simulink model "pidsimu"  (Simulink 6.0)
settings: Solver=ode45  StartTime=0.0  StopTime=60  MaxStep=1  MinStep=0.001  RelTol=1e-2
settings Model: LastModifiedBy=hp  BufferReuse=off
settings SolverCC: InitialStep=0.01
settings DataIOCC: SignalLoggingName=sigsOut  Refine=3
settings OptimizationCC: InlineInvariantSignals=off  OptimizeBlockIOStorage=off  BufferReuse=off  EnforceIntegerDowncast=off  ExpressionFolding=off  FoldNonRolledExpr=off  LocalBlockOutputs=off
settings DebuggingCC: SolverPrmCheckMsg=none
settings HardwareCC: TargetUnknown=on

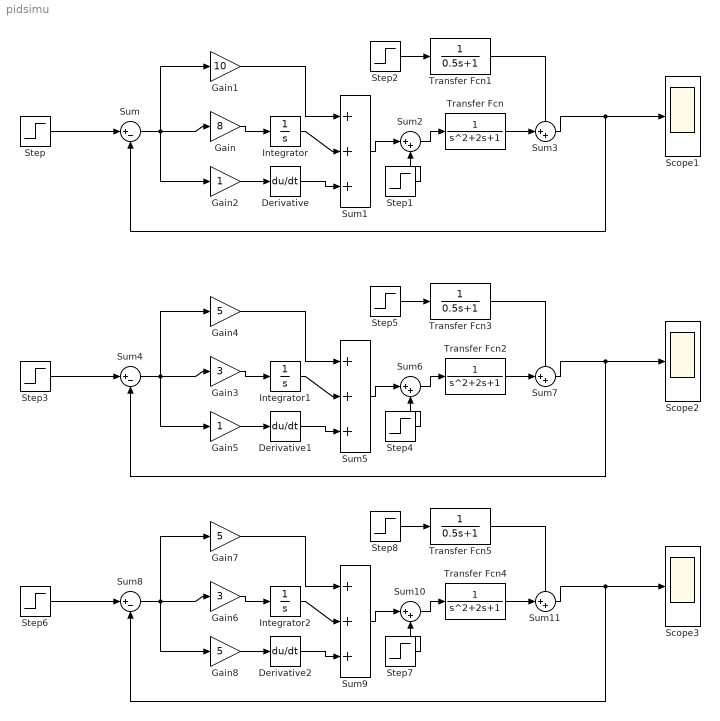
== system pidsimu ==
  Derivative : Derivative
  Derivative1 : Derivative
  Derivative2 : Derivative
  Gain : Gain  Gain=8  SaturateOnIntegerOverflow=on
  Gain1 : Gain  Gain=10  SaturateOnIntegerOverflow=on
  Gain2 : Gain  SaturateOnIntegerOverflow=on
  Gain3 : Gain  Gain=3  SaturateOnIntegerOverflow=on
  Gain4 : Gain  Gain=5  SaturateOnIntegerOverflow=on
  Gain5 : Gain  SaturateOnIntegerOverflow=on
  Gain6 : Gain  Gain=3  SaturateOnIntegerOverflow=on
  Gain7 : Gain  Gain=5  SaturateOnIntegerOverflow=on
  Gain8 : Gain  Gain=5  SaturateOnIntegerOverflow=on
  Integrator : Integrator
  Integrator1 : Integrator
  Integrator2 : Integrator
  Scope1 : Scope
      settings: TimeRange=60  YMin=0  YMax=1.5  SampleInput=on
  Scope2 : Scope
      settings: TimeRange=60  YMin=0  YMax=1.5  SampleInput=on
  Scope3 : Scope
      settings: TimeRange=60  YMin=0  YMax=1.5  SaveName=ScopeData2  SampleInput=on
  Step : Step  Time=0  SampleTime=0.1
  Step1 : Step  Time=20  SampleTime=0.1
  Step2 : Step  Time=40  SampleTime=0.1
  Step3 : Step  Time=0  SampleTime=0.1
  Step4 : Step  Time=20  SampleTime=0.1
  Step5 : Step  Time=40  SampleTime=0.1
  Step6 : Step  Time=0  SampleTime=0.1
  Step7 : Step  Time=20  SampleTime=0.1
  Step8 : Step  Time=40  SampleTime=0.1
  Sum : Sum  Inputs=|+-  SaturateOnIntegerOverflow=on
  Sum1 : Sum  Inputs=|+++  SaturateOnIntegerOverflow=on
  Sum{2..3,6..7,10..11} (6 alike) : Sum  Inputs=|++  SaturateOnIntegerOverflow=on
  Sum4 : Sum  Inputs=|+-  SaturateOnIntegerOverflow=on
  Sum5 : Sum  Inputs=|+++  SaturateOnIntegerOverflow=on
  Sum8 : Sum  Inputs=|+-  SaturateOnIntegerOverflow=on
  Sum9 : Sum  Inputs=|+++  SaturateOnIntegerOverflow=on
  Transfer Fcn : TransferFcn  Numerator=[1 ]
  Transfer Fcn1 : TransferFcn  Numerator=[1 ]  Denominator=[ 0.5 1]
  Transfer Fcn2 : TransferFcn  Numerator=[1 ]
  Transfer Fcn3 : TransferFcn  Numerator=[1 ]  Denominator=[ 0.5 1]
  Transfer Fcn4 : TransferFcn  Numerator=[1 ]
  Transfer Fcn5 : TransferFcn  Numerator=[1 ]  Denominator=[ 0.5 1]
  wires:
  Step/1 -> Sum/1
  Sum/1 -> Gain/1, Gain2/1, Gain1/1
  Gain1/1 -> Sum1/1
  Gain/1 -> Integrator/1
  Integrator/1 -> Sum1/2
  Gain2/1 -> Derivative/1
  Derivative/1 -> Sum1/3
  Sum1/1 -> Sum2/1
  Sum2/1 -> Transfer Fcn/1
  Step1/1 -> Sum2/2
  Step2/1 -> Transfer Fcn1/1
  Transfer Fcn/1 -> Sum3/1
  Sum3/1 -> Scope1/1, Sum/2
  Transfer Fcn1/1 -> Sum3/2
  Step3/1 -> Sum4/1
  Sum4/1 -> Gain3/1, Gain5/1, Gain4/1
  Gain4/1 -> Sum5/1
  Gain3/1 -> Integrator1/1
  Integrator1/1 -> Sum5/2
  Gain5/1 -> Derivative1/1
  Derivative1/1 -> Sum5/3
  Sum5/1 -> Sum6/1
  Sum6/1 -> Transfer Fcn2/1
  Step4/1 -> Sum6/2
  Step5/1 -> Transfer Fcn3/1
  Transfer Fcn2/1 -> Sum7/1
  Sum7/1 -> Scope2/1, Sum4/2
  Transfer Fcn3/1 -> Sum7/2
  Step6/1 -> Sum8/1
  Sum8/1 -> Gain6/1, Gain8/1, Gain7/1
  Gain7/1 -> Sum9/1
  Gain6/1 -> Integrator2/1
  Integrator2/1 -> Sum9/2
  Gain8/1 -> Derivative2/1
  Derivative2/1 -> Sum9/3
  Sum9/1 -> Sum10/1
  Sum10/1 -> Transfer Fcn4/1
  Step7/1 -> Sum10/2
  Step8/1 -> Transfer Fcn5/1
  Transfer Fcn4/1 -> Sum11/1
  Sum11/1 -> Scope3/1, Sum8/2
  Transfer Fcn5/1 -> Sum11/2
